simulink model "HavelZap3"  (Simulink 8.2)
settings: Solver=ode45  StartTime=0.0  StopTime=10.0  RelTol=1e-3
settings Model: Creator=Vojta  LastModifiedBy=Vojta
settings DataIOCC: SignalLoggingSaveFormat=Dataset
settings OptimizationCC: ExpressionDepthLimit=128
settings DebuggingCC: FcnCallInpInsideContextMsg=EnableAllAsError  StateNameClashWarn=none
settings GRTTargetCC: CombineOutputUpdateFcns=on  GRTInterface=off

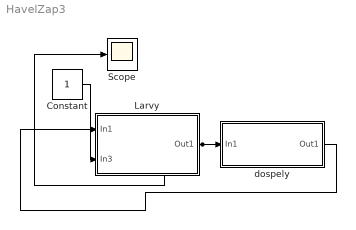
== system HavelZap3 ==
  Constant : Constant
  Larvy : Subsystem
  Scope : Scope
  dospely : Subsystem
  wires:
  Larvy/1(Out1) -> Scope/1, dospely/1(In1)
  dospely/1(Out1) -> Larvy/1(In1)
  Constant/1 -> Larvy/2(In3)

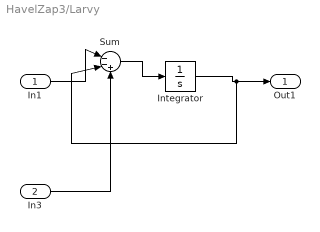
== system HavelZap3/Larvy ==
  In1 : Inport
  In3 : Inport  Port=2
  Integrator : Integrator
  Sum : Sum  Inputs=|--+
  Out1 : Outport
  wires:
  Integrator/1 -> Sum/2, Out1/1
  In1/1 -> Sum/1
  Sum/1 -> Integrator/1
  In3/1 -> Sum/3

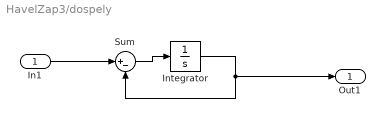
== system HavelZap3/dospely ==
  In1 : Inport
  Integrator : Integrator
  Sum : Sum  Inputs=|+-
  Out1 : Outport
  wires:
  In1/1 -> Sum/1
  Integrator/1 -> Sum/2, Out1/1
  Sum/1 -> Integrator/1
